simulink model "Simulacion_stepper_2024a"  (R2024a)
settings: Solver=ode4  StartTime=0.0  StopTime=Time_simulation  FixedStep=1/frecuency_simulation  RelTol=1e-3
InitFcn:
  | %%InitFcn();
StopFcn:
  | %%FinishFcn
model workspace (MAT data in the model file):
  Ts_stepper = 0.001
values from neighbouring files (symbols this model uses):
  B = motor_params.B_internal    [bode.m]    (also in current_observer.m = 0.0005; discretizacion.m = [ 1/L, 0; ekf_4_estados.m = params.B; obs_ctrl_back_emf_ext.m = [1/L 0)
  B0 = 3*wn_w - BJ_hat    [Barrido_B.m]    (also in Barrido_J.m; InitFcn.m = 449.962302294)
  B1 = 3*wn_w^2 - B0*BJ_hat    [Barrido_B.m]    (also in Barrido_J.m; InitFcn.m = 64448.3670019)
  B2 = -(J_var/P)*(wn_w^3)    [Barrido_B.m]    (also in Barrido_J.m; InitFcn.m = -0.364323750994)
  B_internal = 1e-4    (= 0.0001)    [InitFcn.m]
  B_var = B_internal* B_factors(k)    [Barrido_B.m]    (also in Barrido_J.m = B_real; InitFcn.m = 0.0001)
  frecuency_simulation = 10e3    (= 10000)    [InitFcn.m]
  I_nom = 1    [InitFcn.m]    (also in salient_motor.m)
  J = motor_params.J_internal    [bode.m]    (also in current_observer.m = 0.008; ekf_4_estados.m = params.J; obs_ctrl_back_emf_ext.m = 0.008; obs_y_contrl_back_emd.m = 0.008)
  J_internal = 4.7/1000000    (= 4.7e-06)    [InitFcn.m]
  J_var = J_real    [Barrido_B.m]    (also in Barrido_J.m = J_internal * J_factors(k); InitFcn.m = 4.7e-06)
  Ke = Kt    [InitFcn.m]    (also in current_observer.m = 0.0055; ekf_4_estados.m = params.Ke; observer.m = Pvec(3); salient_motor.m = 0.0066)
  Ki_d = wd_d*R    (= 3926.99081699)    [InitFcn.m]    (also in bode.m = PI_dq_params.Ki_d_salient)
  Ki_d_salient = wd_d^2*Ld    (= 21491.0635834)    [InitFcn.m]
  Ki_q = wd_q*R    (= 3926.99081699)    [InitFcn.m]    (also in bode.m = PI_dq_params.Ki_q_salient)
  Ki_q_salient = wd_q^2*Lq    (= 7846.33549887)    [InitFcn.m]
  Ki_w = (wn_w^2)*J_var/Kt    [Barrido_B.m]    (also in Barrido_J.m; InitFcn.m; bode.m = PI_MTPA_params.Ki_w)
  Kp_d = wd_d*L    (= 9.42477796077)    [InitFcn.m]    (also in bode.m = PI_dq_params.Kp_d_salient)
  Kp_d_salient = 2*shi_d*wd_d*Ld -R    (= 16.845833313)    [InitFcn.m]
  Kp_q = wd_q*L    (= 9.42477796077)    [InitFcn.m]    (also in bode.m = PI_dq_params.Kp_q_salient)
  Kp_q_salient = 2*shi_q*wd_q*Lq-R    (= 4.56311709936)    [InitFcn.m]
  Kp_w = (2*shi_w*wn_w*J_var)/Kt    [Barrido_B.m]    (also in Barrido_J.m; InitFcn.m; bode.m = PI_MTPA_params.Kp_w)
  Kt = Thold / (sqrt(2) * I_nom)    [InitFcn.m]    (also in current_observer.m = 0.275; ekf_4_estados.m = params.Kt; frecuencia_max.m = 0.33; observer.m = Pvec(4))
  L = 6/1000    (= 0.006)    [InitFcn.m]    (also in current_observer.m = place(A', C', 10*eig(A)).'; desfase.m = lags(k); discretizacion.m = 0.01; frecuencia_max.m)
  Ld = L0 + L2    [Copy_of_PMSM_salient.m]    (also in InitFcn.m = 0.00871; bode.m = motor_params.Ld; ekf_4_estados.m = params.Ld; salient_motor.m = 0.00871)
  Lq = L0 - L2    [Copy_of_PMSM_salient.m]    (also in InitFcn.m = 0.00318; bode.m = motor_params.Lq; ekf_4_estados.m = params.Lq; salient_motor.m = 0.00318)
  N_steps = 360/Step_angle    (= 200)    [InitFcn.m]
  P = N_teeths/2    (= 50)    [InitFcn.m]    (also in bode.m = motor_params.P; ekf_4_estados.m = P_pred; frecuencia_max.m; salient_motor.m)
  Phi = pi/2    (= 1.57079632679)    [InitFcn.m]    (also in ekf_4_estados.m = eye(4) + Ts_eff*A)
  Psi = Kt/P    [InitFcn.m]    (also in bode.m = motor_params.Ke; salient_motor.m = 0.0066)
  R = 2.5    [InitFcn.m]    (also in bode.m = motor_params.R; current_observer.m = 3.4; discretizacion.m = 3.4; ekf_4_estados.m = params.R)
  sample_time = 1/frecuency_simulation    (= 0.0001)    [InitFcn.m]
  Tdm = 18/1000    (= 0.018)    [InitFcn.m]    (also in salient_motor.m)
  Ts_current = 1/f_current    (= 0.0001)    [InitFcn.m]
  Ts_DO = Ts_Wm    (= 0.0001)    [InitFcn.m]
  Ts_ekf = 1/f_ekf    (= 0.0001)    [InitFcn.m]
  Ts_Wm = Ts_current    (= 0.0001)    [InitFcn.m]
  Vdc = 12    [InitFcn.m]    (also in frecuencia_max.m)
undefined symbols (not defined in the file or in its folder): DiscIntNeverNeededParam
libraries: fl_lib x27, nesl_utility x19, spsMosfetLib x16, simulink x8, eeTransforms x4, spsDCVoltageSourceLib x4, spsVoltageMeasurementLib x4, ee_lib x3, slexportprevious_tp74def212_4eb8_4616_a2bc_f4e795655e99 x1, spsTriangleGeneratorLib x1, spspowerguiLib x1
(part 4 of 4)

== matlab function Simulacion_stepper_2024a/Triggered Subsystem7/MATLAB Function ==
  data: Wm input; Vd output; X input; Theta_e input; Ts input; Vdc input; Kp_d input; Ki_d input; Kp_q input; Ki_q input; Ke input; Ld input; Lq input; P input; Vq output; Id output; Iq output; Iq_ref input
function [Vd, Vq, Id, Iq] = PI_dq( ...
    Wm, X, Theta_e, Ts, Vdc, ...
    Kp_d, Ki_d, Kp_q, Ki_q, ...
    Ke, Ld, Lq, P, Iq_ref) % Limpieza de entradas innecesarias

% ================== Estados del Integrador ==================
persistent ek_d u_d ek_q u_q

% Inicialización única
if isempty(u_d)
    u_d = 0; ek_d = 0;
    u_q = 0; ek_q = 0;
end

%% ================== Transformada de Park (abc/ab -> dq) ==================
% X(1) = Ia, X(2) = Ib (Asumiendo motor bifásico/stepper)
Ia = X(1); Ib = X(2);
C = cos(Theta_e); S = sin(Theta_e);

Id =  Ia*C + Ib*S;
Iq = -Ia*S + Ib*C;

%% ================== Desacoples (Feedforward de Corriente) ==================
We = P * Wm;
% V_compensa = Voltaje que el PI no tiene que "esforzarse" en generar
Vdec_d = -Lq * We * Iq;            % Cruce de eje Q sobre D
Vdec_q = (Ke * Wm) + (Ld * We * Id); % Back-EMF + Cruce de eje D sobre Q

%% ================== PI Incremental Eje Q (Torque) ==================
ek_curr_q = Iq_ref - Iq;
k1_q = Kp_q + Ki_q*Ts;
k2_q = -Kp_q;

du_q = k1_q * ek_curr_q + k2_q * ek_q;
u_q  = u_q + du_q;

%% ================== PI Incremental Eje D (Flujo, ref=0) ==================
ek_curr_d = 0 - Id; % Id_ref es siempre 0 para máxima eficiencia
k1_d = Kp_d + Ki_d*Ts;
k2_d = -Kp_d;

du_d = k1_d * ek_curr_d + k2_d * ek_d;
u_d  = u_d + du_d;

%% ================== Salida + Saturación Circular + Anti-Windup ==================
Vd = u_d + Vdec_d;
Vq = u_q + Vdec_q;

Vnorm = sqrt(Vd^2 + Vq^2);

if Vnorm > Vdc
    scale = Vdc / Vnorm;
    Vd = Vd * scale;
    Vq = Vq * scale;
    
    % Anti-windup incremental: "congelamos" la integral restando el exceso
    u_d = Vd - Vdec_d;
    u_q = Vq - Vdec_q;
else
    % Solo actualizamos errores previos si no hubo saturación
    ek_d = ek_curr_d;
    ek_q = ek_curr_q;
end

end

== matlab function Simulacion_stepper_2024a/Triggered Subsystem8/MATLAB Function ==
  data: Wm_ref input; Wm input; Ts input; Kp_w input; Ki_w input; Tl_tdm input; B input; Kt input; Imax input; Iq_ref output
function Iq_ref = PI_speed( ...
        Wm_ref, Wm, Ts, ...
        Kp_w, Ki_w, ...
        Tl_tdm, B, Kt, ...
        Imax)
% ================== Estados del Integrador ==================
persistent ek_w u_w
% Inicialización única al arrancar la simulación
if isempty(u_w)
    u_w  = 0;
    ek_w = 0; 
end

% ================== Feedforward (Modelo de la Planta) ==================
% Torque base necesario para compensar carga y roce viscoso
Iq_ff = (Tl_tdm + B*Wm)/Kt;

% ================== PI incremental ==================
% Error actual
ek_curr = Wm_ref - Wm;

% Constantes del controlador incremental
k1_w = Kp_w + Ki_w*Ts;
k2_w = -Kp_w;

% Cálculo del incremento de control (du) y actualización de la integral (u)
% du = Kp*(ek - ek_prev) + Ki*Ts*ek
du_w = k1_w * ek_curr + k2_w * ek_w;
u_w  = u_w + du_w;

% La referencia final es el aporte del PI + el Feedforward de la planta
Iq_ref = Iq_ff + u_w;

% ================== Saturación con Anti-Windup ==================
if abs(Iq_ref) > Imax
    Iq_ref = sign(Iq_ref) * Imax;
    % Detenemos la integración: restamos el incremento para "congelar" u_w
    u_w = u_w - du_w;
else
    % Solo actualizamos el error previo si no estamos saturados
    % (o puedes actualizarlo siempre, según prefieras el comportamiento del transitorio)
    ek_w = ek_curr;
end

end

== matlab function Simulacion_stepper_2024a/MATLAB Function5 ==
  data: u input; y output
function y = fcn(u)

y = wrap_2pi(u);

== matlab function Simulacion_stepper_2024a/MATLAB Function11 ==
  data: u input; y output
function y = fcn(u)

y = wrap_2pi(u);

== matlab function Simulacion_stepper_2024a/MATLAB Function8 ==
  data: u input; y output
function y = fcn(u)

y = wrap_2pi(u);

== matlab function Simulacion_stepper_2024a/Triggered Subsystem10/MATLAB Function ==
  data: Wm_ref input; Wm input; Ts input; Kp_w input; Ki_w input; Tl_tdm input; B input; Kt input; theta_e input; Tdm input; Imax input; Iq_ref output; Wm_filt_out output
function [Iq_ref,Wm_filt_out] = PI_speed( ...
        Wm_ref, Wm, Ts, ...
        Kp_w, Ki_w, ...
        Tl_tdm, B, Kt, theta_e, Tdm, ...
        Imax)

% ================== Estados Persistentes ==================
% Añadimos Wm_filt para guardar el estado del filtro
persistent ek_w u_w Wm_filt
if isempty(u_w)
    u_w  = 0;
    ek_w = 0; 
    Wm_filt = Wm; % Inicializamos el filtro con el primer valor medido
end

% ================== Filtro Pasabajos (LPF) ==================
% Definimos la frecuencia de corte del filtro (fc). 
% Para un BW de velocidad de 20Hz, un fc de 50-100Hz es ideal.
%  fc = 150; 
%  tau = 1/(2*pi*fc);
% alpha = tau/(tau + Ts); % Coeficiente del filtro
% % 
% % % Aplicamos el filtro a la velocidad medida
%  Wm_f = alpha * Wm_filt + (1 - alpha) * Wm;
%  Wm_filt = Wm_f; % Actualizamos el estado para la próxima iteración

% ================== Feedforward (Modelo de la Planta) ==================
% Es mejor usar la velocidad filtrada para el término viscoso
Iq_ff = (Tl_tdm + B*Wm)/Kt;
Iq_cogging = 0;%% (Tdm * sin(4 * theta_e)) / Kt;
% ================== PI incremental ==================
% El error ahora se calcula con la velocidad FILTRADA
ek_curr = Wm_ref - Wm;

k1_w = Kp_w + Ki_w*Ts;
k2_w = -Kp_w;

du_w = k1_w * ek_curr + k2_w * ek_w;
u_w  = u_w + du_w;

% La referencia final
Iq_ref = -Iq_ff + u_w + Iq_cogging;
Wm_filt_out = Wm_filt;
% ================== Saturación con Anti-Windup ==================
if abs(Iq_ref) > Imax
    Iq_ref = sign(Iq_ref) * Imax;
    u_w = u_w - du_w;
else
    ek_w = ek_curr;
end

end

== matlab function Simulacion_stepper_2024a/Triggered Subsystem2/MATLAB Function ==
  data: U input; x_corr output; X input; Ts input; Ke input; Kt input; R input; J input; Ld input; Lq input; Nr input; B input; Te_est output; Tdm input
function [x_corr, Te_est] = ekf_dq_4states_final(U, X, Ts, Ke, Kt, R, J, Ld, Lq, Nr, B, Tdm)
% =========================================================================
% EKF DE 4 ESTADOS: [Id; Iq; Wm; Th_m]
% =========================================================================
% Entradas:
%   U   = [Vd; Vq]            -> Tensiones de control
%   X   = [Ia; Ib; Theta_e_m] -> Corrientes y Ángulo HFI (Medidos)
%   Ts  = Tiempo de muestreo
% =========================================================================
persistent x_hat P
if isempty(x_hat)
    x_hat = zeros(4,1); 
    % P inicial (4x4)
    P = diag([1e-4, 1e-4, 1e-2, 1e-4]);
end

% -------------------------------------------------------------------------
% 1. TRANSFORMADA DE PARK (Entrada de mediciones)
% -------------------------------------------------------------------------
Ia = X(1); Ib = X(2); The_e_m = X(3);
cos_th = cos(The_e_m);
sin_th = sin(The_e_m);

% Park Directa para obtener corrientes en marco dq medido
Id_m =  Ia * cos_th + Ib * sin_th;
Iq_m = -Ia * sin_th + Ib * cos_th;

Vd_m =  U(1) * cos_th + U(2) * sin_th;
Vq_m = -U(1) * sin_th + U(2) * cos_th;

% -------------------------------------------------------------------------
% 2. PREDICCIÓN (MODELO DE 4 ESTADOS)
% -------------------------------------------------------------------------
Id = x_hat(1); Iq = x_hat(2); Wm = x_hat(3); Th_m = x_hat(4);

% Ecuaciones dinámicas f(x,u)
dId = (Vd_m - R*Id + Nr*Wm*Lq*Iq) / Ld;
dIq = (Vq_m - R*Iq - Nr*Wm*Ld*Id - Ke*Wm) / Lq;
Te  = Kt*Iq + (Ld - Lq)*Id*Iq; % Torque total
% Nota: Aquí eliminamos Tx. El torque de carga ahora se trata como ruido de proceso.
dWm = (Te - B*Wm - Tdm*sin(4*Nr*Th_m)) / J; 
dTh = Wm;

% Predicción de estado (Integración de Euler)
x_pred = x_hat + Ts * [dId; dIq; dWm; dTh];
x_pred(4) = wrap_pi(x_pred(4));

% -------------------------------------------------------------------------
% 3. LINEALIZACIÓN (JACOBIANO A DE 4x4)
% -------------------------------------------------------------------------
A = [ -R/Ld,                Nr*Wm*Lq/Ld,         Nr*Lq*Iq/Ld,         0;
     -Nr*Wm*Ld/Lq,         -R/Lq,               -(Nr*Ld*Id + Ke)/Lq,  0;
      (Ld-Lq)*Iq/J,     (Kt + Nr*(Ld-Lq)*Id)/J, -B/J,              0;
      0,                   0,                   1,                    0];
    
Phi = eye(4) + A*Ts;

% Covarianza del proceso Qk (4x4)
% Al no estimar Tx, es vital que Qk(3,3) sea un poco más alto para absorber
% las variaciones de carga como incertidumbre en la velocidad.
Qk = diag([1e-6, 1e-6, 1e-6, 1e-10]); 
P_pred = Phi * P * Phi' + Qk;

% -------------------------------------------------------------------------
% 4. CORRECCIÓN (INNOVACIÓN Y GANANCIA)
% -------------------------------------------------------------------------
% Matriz de observación Ck (Medimos Id, Iq y Theta_e_m -> Nr * Th_m)
Ck = [1 0 0 0;
      0 1 0 0;
      0 0 0 Nr]; 

% Ruido de medición
Rk = diag([1e-3, 1e-3, 1e-8]);

y_meas = [Id_m; Iq_m; The_e_m];
y_pred = [x_pred(1); x_pred(2); Nr * x_pred(4)];

innov = y_meas - y_pred;
innov(3) = wrap_pi(innov(3));

% Ganancia de Kalman
Sk = Ck * P_pred * Ck' + Rk;
Lk = (P_pred * Ck') / Sk; % Lk es ahora de 4x3

% Actualización de estado y covarianza
x_corr = x_pred + Lk * innov;
x_corr(4) = wrap_pi(x_corr(4));

P = (eye(4) - Lk*Ck) * P_pred;
P = 0.5 * (P + P'); % Asegurar simetría

% -------------------------------------------------------------------------
% 5. PERSISTENCIA Y SALIDAS
% -------------------------------------------------------------------------
x_hat = x_corr;
Te_est = Kt*x_corr(2) + (Ld-Lq)*x_corr(1)*x_corr(2);

end

function out = wrap_pi(in)
    out = atan2(sin(in), cos(in));
end

== matlab function Simulacion_stepper_2024a/Triggered Subsystem2/MATLAB Function1 ==
  data: U input; x_corr output; X input; Ts input; Kt input; R input; J input; L input; Nr input; B input; Ke input
function x_corr = ekf_5var(U,X,Ts,Kt,R,J,L,Nr,B,Ke)
persistent x_hat P x_pred
%%  x_hat son los estados predichos
%%  x_corr es la salida corregida
%%  P_pre ó Sum_less es la covarianza predicha
%%  P ó sum_more es la covarianza
%%  Rk ó sum_v es la covarianza de incertidumbre del sensor




 %%Iniciamos calculando X_hat[k-1]
 if isempty(x_hat)
     x_hat = zeros(5,1);
     P = diag([1e-4 1e-4 1e-6 1e-10 1e-4]);
     x_corr = zeros(5,1);
     x_pred = zeros(5,1);


 end

Qk = diag([1e-4 1e-4 1e-4 1e-10 1e-6]);
Rk = diag([5e-4 5e-4]);   % ruido de medición

%%1A
%%Predicción
Ia = x_hat(1);
Ib = x_hat(2);
Wm = x_hat(3);
Th_m = x_hat(4);
Tx = x_hat(5);

Th_e = Nr*Th_m;
S = sin(Th_e);
C = cos(Th_e);

Va = U(1);
Vb = U(2);

dx = zeros(5,1);
dx(1) = (Va - R*Ia + Ke*Wm*S)/L;
dx(2) = (Vb - R*Ib - Ke*Wm*C)/L;
dx(3) = (Kt*(Ib*C-Ia*S) -Tx)/J;
dx(4) = Wm;
dx(5) = 0;
x_pred = x_hat + Ts*dx;
x_pred(4) = wrap_2pi(x_pred(4));

%%Calculamos el jacobiano
RL = R/L;
uno = Ke*S;
dos = Ke*C;

A = [-RL 0   (uno/L) (dos*Nr*Wm/L) 0;
 0  -RL   -dos/L    uno*Nr*Wm/L  0;
 -uno/J dos/J -1/J -Kt*Nr*(Ia*C+Ib*S)/J -1/J;
 0 0 1 0 0;
 0 0 0 0 0];

A_hat = eye(5) + Ts*A;
A_hat_T = transpose(A_hat);

%%1B COVARIANZA PREDICHA
P_pred = A_hat * P * A_hat_T + Qk; 


%%1C PREDECIMOS LA SALIDA DEL SISTEMA
Ck = [1 0 0 0 0;
      0 1 0 0 0];
Ck_T = transpose(Ck);
y_pred = Ck*x_pred;

%%2A calculamos la matriz Lk
%%Lk = P_pred *Ck_T * inv(Ck*P_pred*Ck_T + sum_v)
Sk = Ck*P_pred*Ck_T + Rk;
Lk = P_pred * Ck_T /Sk;

%%2B Actualizamos los estados estados corregidos en función de L


y_meas = [X(1);X(2)];

innov = y_meas - y_pred;
x_corr = x_pred + Lk*(innov);
x_corr(4) = wrap_2pi(x_corr(4));
%%actualizamos la covarianza y guardamos el estado
x_hat = x_corr;
Lk_T = transpose(Lk);
P = P_pred - Lk*Sk*Lk_T;
P_T = transpose(P);
P = 0.5 * (P + P_T);

== matlab function Simulacion_stepper_2024a/Triggered Subsystem2/MATLAB Function2 ==
  data: U input size=2; x_corr output; Y input size=2; Ts input; Kt input; R input; J input; L input; Nr input; B input
function x_corr = SPKF_4var(U,Y,Ts,Kt,R,J,L,Nr,B)
persistent x_hat P  alpham alphac Qk Rk h
%%  x_hat son los estados predichos
%%  x_corr es la salida corregida
%%  P_pre ó Sum_less es la covarianza predicha
%%  P ó sum_more es la covarianza
%%  Rk ó sum_v es la covarianza de incertidumbre del sensor


Nx = 4; %%Números de estados
Nw = 4; %% Incertidumbres de estado
Ny = 2; %% Incertidumbre de mediciones
Na = Nx+Nw+Ny;


%%Los métodos de sigma-point pueden diferir al utilizar las variables
%%alpha. Existen 2 métodos:

%% Método |    Sigma       |     alpha_m_0      | alpha_m_k         |           alpha_c_0               | alpha_c_k |
%% UKF    | sqrt(L+lambda) |  lambda/(L+Lambda) | 1/(2*(L+Lambda))  | alpha_m_0 + (1-alpha^2 + betha)   | alpha_m_k |
%% CDKF   |    h           |   (h^2 - L)/h^2    |  1/(2*h^2)        | alpha_m_0                         | alpha_m_k |
 %%Iniciamos calculando X_hat[k-1]
 if isempty(x_hat)
    
     %%Utilizamos el CDKF, con h = sqrt(Nxa); 
        x_hat = zeros(Nx,1);
        h =sqrt(Na);
        alpham = ones(2*Na+1,1) * (1/(2*h^2));
        alpham(1) = (h^2 - Na)/(h^2);   % peso del sigma central
        alphac = alpham;             
     %%Valores de covarianza
     P = diag([1e-2 1e-2 1e-6 1e-12 ]);
     Qk = diag([1e-2 1e-2 1e-8 1e-12 ]);
     Rk = [1e-4 0; 0 1e-4];
 end
    
     x_corr = zeros(Nx,1);
     x_pred = zeros(Nx,1);
     x_hat_a = zeros(Na,1);
     X_minus = zeros(Nx,2*Na+1);
     Y_minus = zeros(Ny,2*Na+1);
%%Ciclo de 2*Na+1
%%Aun que deberiamos hacer un ciclo for, en matlab se hace solo asi que no
%%es necesario

%% 1A-I Creamos el vector de estados extendidos
x_hat_a = [x_hat;zeros(Nw,1);zeros(Ny,1)]; 


%% 1A-II Conseguimos el factor de cholesky


%%Creamos la matriz de covarianza extendidas, el cual es de la forma
%%             [P   0    0]
%%     P_a =   [0   Qk   0]
%%             [0   0   Rk]

P_a = blkdiag(P,Qk,Rk);
Sa = chol(P_a,"lower");

%% 1A-III generamos los sigma points
%% Queda de la forma [x_hat_a, x_hat_a + h*S,x_hat_a - h*S] (Por eso es 2*Nxa+1 = N)
%% Al usar x_a x_a(:,ones(1,Na)) creamos una matriz de la forma [x_a,x_a...x_a], que es de tamaño (Na)x(2*Na+1)
%% Posteriormente, se le suma un vector de [0,+h*S,-h*S]
%% Cómo S es del tamaño (Nxa)x(Nxa), el total es de (2*Na+1 = N)
X =  x_hat_a(:,ones(1,2*Na+1)) + h*[zeros(Na,1), Sa, -Sa];

%% 1A-IV Calculamos las ecuaciones de estado
Va = U(1);
Vb = U(2);


for k=1:2*Na+1

  % --- separar estado, ruido de proceso y ruido de medición ---


xk = X(1:Nx,k);                     % [Ia; Ib; Wm; Th_m]
wk = X(Nx+1 : Nx+Nw,k);             % ruido de proceso (4x1)
vk = X(Nx+Nw+1 : end,k);            % ruido de medición (2x1)    

Ia = xk(1);
Ib = xk(2);
Wm = xk(3);
Th_m = xk(4);

Th_e = Nr*Th_m;
S = sin(Th_e);
C = cos(Th_e);


dx1 = (Va - R*Ia + Kt*Wm*S)/L;
dx2 = (Vb - R*Ib - Kt*Wm*C)/L;
dx3 = (Kt*(Ib*C-Ia*S)-B*Wm)/J;
dx4 = Wm;

%Calculamos el paso siguiente mediante euler
%% X_minus corresponde a la matriz que contiene todos los sigma-points distribuidos en los estados del sistema no-extendido (Nx)x(Na)
X_minus(1,k) = Ia + Ts*dx1+ wk(1);
X_minus(2,k) = Ib + Ts*dx2 + wk(2);
X_minus(3,k) = Wm + Ts*dx3 + wk(3);
X_minus(4,k) = Th_m + Ts*dx4 + wk(4);
%%X_minus(4,k) = wrap_2pi(X_minus(4,k));

Y_minus(1,k) = X_minus(1,k) + vk(1);
Y_minus(2,k) = X_minus(2,k) + vk(2);

end
%% 1B Reconstrucción de la media
%% Esta matriz contiene la media de todos los estados. (Nx)x(1)
x_pred = X_minus*alpham;
y_pred = Y_minus*alpham;
%%  Reconstrucción de la covarianza

%% Acá lo que hacemos es copiar la media N veces, para poder realizar la resta.
%%Pero realmente debería ser un for de [Xs(i,k)= X_minus(i,k) - x_pred(i)],
%%dónde K es cada variable de estado (Nx)
%% Xs es una matriz de desviación respecto a la media. Es necesario para construir la covarianza P
Xs = X_minus - x_pred(:,ones([1 2*Na+1])); 
Ys = Y_minus - y_pred(:,ones([1 2*Na+1]));

Xs_T = transpose(Xs);
Ys_T = transpose(Ys);
%%Calculamos la matriz de covarianza, pero hay que considerar que como
%%diag(alphac) es una matriz llena de diagonales, uno puede reducir la
%%cantidad de cómputo.
P_pred = Xs*diag(alphac)*Xs_T;
Pyy = Ys* diag(alphac)* Ys_T;
Pxy = Xs*diag(alphac)*Ys_T;
Lk = Pxy/Pyy;
Lk_T = transpose(Lk);
%% 2B Leemos la medición y actualizamos
x_corr = x_pred + Lk*(Y - y_pred);
x_corr(4) = wrap_2pi(x_corr(4));
%%Guardamos los valores de x_hat para mantenerlos
x_hat = x_corr; 
%% 2C Actualizamos la covarianza
P = P_pred - Lk*Pyy*Lk_T;
P_T = transpose(P);
P = 0.5 * (P + P_T);

== matlab function Simulacion_stepper_2024a/Triggered Subsystem2/MATLAB Function3 ==
  data: U input size=2; x_corr output; Y input size=2; Ts input; Kt input; R input; J input; L input; Nr input; B input
function x_corr = SPKF_5var(U,Y,Ts,Kt,R,J,L,Nr,B)
persistent x_hat P x_pred alpham alphac Qk Rk h
%%  x_hat son los estados predichos
%%  x_corr es la salida corregida
%%  P_pre ó Sum_less es la covarianza predicha
%%  P ó sum_more es la covarianza
%%  Rk ó sum_v es la covarianza de incertidumbre del sensor


Nx = 5; %%Números de estados
Nw = 5; %% Incertidumbres de estado
Ny = 2; %% Incertidumbre de mediciones
Na = Nx+Nw+Ny;


%%Los métodos de sigma-point pueden diferir al utilizar las variables
%%alpha. Existen 2 métodos:

%% Método |    Sigma       |     alpha_m_0      | alpha_m_k         |           alpha_c_0               | alpha_c_k |
%% UKF    | sqrt(L+lambda) |  lambda/(L+Lambda) | 1/(2*(L+Lambda))  | alpha_m_0 + (1-alpha^2 + betha)   | alpha_m_k |
%% CDKF   |    h           |   (h^2 - L)/h^2    |  1/(2*h^2)        | alpha_m_0                         | alpha_m_k |
 %%Iniciamos calculando X_hat[k-1]
 if isempty(x_hat)
    
     %%Utilizamos el CDKF, con h = sqrt(Nxa); 
        x_hat = zeros(Nx,1);
        h =sqrt(Na);
        alpham = ones(2*Na+1,1) * (1/(2*h^2));
        alpham(1) = (h^2 - Na)/(h^2);   % peso del sigma central
        alphac = alpham;             
     %%Valores de covarianza
     P = diag([1e-2 1e-2 1e-4 1e-8 1e-12]);
     Qk = diag([1e-2 1e-2 1e-6 1e-8 1e-12]);
     Rk = [1e-4 0; 0 1e-4];
 end
    
     x_corr = zeros(Nx,1);
     x_pred = zeros(Nx,1);
     x_hat_a = zeros(Na,1);
     X_minus = zeros(Nx,2*Na+1);
     Y_minus = zeros(Ny,2*Na+1);
%%Ciclo de 2*Na+1
%%Aun que deberiamos hacer un ciclo for, en matlab se hace solo asi que no
%%es necesario

%% 1A-I Creamos el vector de estados extendidos
x_hat_a = [x_hat;zeros(Nw,1);zeros(Ny,1)]; 


%% 1A-II Conseguimos el factor de cholesky


%%Creamos la matriz de covarianza extendidas, el cual es de la forma
%%             [P   0    0]
%%     P_a =   [0   Qk   0]
%%             [0   0   Rk]

P_a = blkdiag(P,Qk,Rk);
Sa = chol(P_a,"lower");

%% 1A-III generamos los sigma points
%% Queda de la forma [x_hat_a, x_hat_a + h*S,x_hat_a - h*S] (Por eso es 2*Nxa+1 = N)
%% Al usar x_a x_a(:,ones(1,Na)) creamos una matriz de la forma [x_a,x_a...x_a], que es de tamaño (Na)x(2*Na+1)
%% Posteriormente, se le suma un vector de [0,+h*S,-h*S]
%% Cómo S es del tamaño (Nxa)x(Nxa), el total es de (2*Na+1 = N)
X =  x_hat_a(:,ones(1,2*Na+1)) + h*[zeros(Na,1), Sa, -Sa];

%% 1A-IV Calculamos las ecuaciones de estado
Va = U(1);
Vb = U(2);


for k=1:2*Na+1

  % --- separar estado, ruido de proceso y ruido de medición ---


xk = X(1:Nx,k);                     % [Ia; Ib; Wm; Th_m]
wk = X(Nx+1 : Nx+Nw,k);             % ruido de proceso (4x1)
vk = X(Nx+Nw+1 : end,k);            % ruido de medición (2x1)    

Ia = xk(1);
Ib = xk(2);
Wm = xk(3);
Th_m = xk(4);
Tx = xk(5);

Th_e = Nr*Th_m;
S = sin(Th_e);
C = cos(Th_e);


dx1 = (Va - R*Ia + Kt*Wm*S)/L;
dx2 = (Vb - R*Ib - Kt*Wm*C)/L;
dx3 = (Kt*(Ib*C-Ia*S)-B*Wm - Tx)/J;
dx4 = Wm;
dTx = 0;

%Calculamos el paso siguiente mediante euler
%% X_minus corresponde a la matriz que contiene todos los sigma-points distribuidos en los estados del sistema no-extendido (Nx)x(Na)
X_minus(1,k) = Ia + Ts*dx1+ wk(1);
X_minus(2,k) = Ib + Ts*dx2 + wk(2);
X_minus(3,k) = Wm + Ts*dx3 + wk(3);
X_minus(4,k) = Th_m + Ts*dx4 + wk(4);
X_minus(4,k) = wrap_2pi(X_minus(4,k));
X_minus(5,k) = Tx + Ts*dTx + wk(5);

Y_minus(1,k) = X_minus(1,k) + vk(1);
Y_minus(2,k) = X_minus(2,k) + vk(2);

end
%% 1B Reconstrucción de la media
%% Esta matriz contiene la media de todos los estados. (Nx)x(1)
x_pred = X_minus*alpham;
y_pred = Y_minus*alpham;
%%  Reconstrucción de la covarianza

%% Acá lo que hacemos es copiar la media N veces, para poder realizar la resta.
%%Pero realmente debería ser un for de [Xs(i,k)= X_minus(i,k) - x_pred(i)],
%%dónde K es cada variable de estado (Nx)
%% Xs es una matriz de desviación respecto a la media. Es necesario para construir la covarianza P
Xs = X_minus - x_pred(:,ones([1 2*Na+1])); 
Ys = Y_minus - y_pred(:,ones([1 2*Na+1]));

Xs_T = transpose(Xs);
Ys_T = transpose(Ys);
%%Calculamos la matriz de covarianza, pero hay que considerar que como
%%diag(alphac) es una matriz llena de diagonales, uno puede reducir la
%%cantidad de cómputo.
P_pred = Xs*diag(alphac)*Xs_T;
Pyy = Ys* diag(alphac)* Ys_T;
Pxy = Xs*diag(alphac)*Ys_T;
Lk = Pxy/Pyy;
Lk_T = transpose(Lk);
%% 2B Leemos la medición y actualizamos
x_corr = x_pred + Lk*(Y - y_pred);
x_corr(4) = wrap_2pi(x_corr(4));
%%Guardamos los valores de x_hat para mantenerlos
x_hat = x_corr; 
%% 2C Actualizamos la covarianza
P = P_pred - Lk*Pyy*Lk_T;
P_T = transpose(P);
P = 0.5 * (P + P_T);

== matlab function Simulacion_stepper_2024a/MATLAB Function9 ==
  data: u input; y output
function y = fcn(u)

y = wrap_2pi(u);

== matlab function Simulacion_stepper_2024a/MATLAB Function10 ==
  data: u input; y output
function y = fcn(u)

y = wrap_2pi(u);

== matlab function Simulacion_stepper_2024a/Triggered Subsystem4/MATLAB Function ==
  data: Wm input; x_corr output; Iq input; Ts input; Kt input; J input
function x_corr = ekf_2var(Wm,Iq,Ts,Kt,J)
persistent x_hat P x_pred
%%  x_hat son los estados predichos
%%  x_corr es la salida corregida
%%  P_pre ó Sum_less es la covarianza predicha
%%  P ó sum_more es la covarianza
%%  Rk ó sum_v es la covarianza de incertidumbre del sensor




 %%Iniciamos calculando X_hat[k-1]
 if isempty(x_hat)
     x_hat = zeros(2,1);
     P = diag([1e-5 1e-3 ]);
     x_corr = zeros(2,1);
     x_pred = zeros(2,1);


 end

Qk = diag([1e-2 5e-7]);
Rk = diag(5e-1);   % ruido de medición

%%1A
%%Predicción

Wm = x_hat(1);
Tx = x_hat(2);


Te = Iq*Kt;

dx = zeros(2,1);
dx(1) = (Te - Tx)/J;
dx(2) = 0;

x_pred = x_hat + Ts*dx;




A = [0 -1/J; 0 0];

% A_hat = eye(4) + Ts*A;
A_hat = expm(A*Ts);
A_hat_T = transpose(A_hat);

%%1B COVARIANZA PREDICHA
P_pred = A_hat * P * A_hat_T + Qk; 


%%1C PREDECIMOS LA SALIDA DEL SISTEMA
Ck = [1 0];
Ck_T = transpose(Ck);
y_pred = Ck*x_pred;

%%2A calculamos la matriz Lk
%%Lk = P_pred *Ck_T * inv(Ck*P_pred*Ck_T + sum_v)
Sk = Ck*P_pred*Ck_T + Rk;
Lk = P_pred * Ck_T /Sk;

%%2B Actualizamos los estados estados corregidos en función de L


y_meas = Wm;

innov = y_meas - y_pred;
x_corr = x_pred + Lk*(innov);

%%actualizamos la covarianza y guardamos el estado
x_hat = x_corr;
Lk_T = transpose(Lk);
P = P_pred - Lk*Sk*Lk_T;
P_T = transpose(P);
P = 0.5 * (P + P_T);

== matlab function Simulacion_stepper_2024a/MATLAB Function12 ==
  data: u input; y output
function y = fcn(u)

y = wrap_2pi(u);

== matlab function Simulacion_stepper_2024a/Triggered Subsystem4/MATLAB Function1 ==
  data: theta_EKF input; Iq_obs input; Ts input; Kt input; np input; J input; theta_hat output; omega_hat output; d_hat output; B input; beta0 input; beta1 input; beta2 input
function [theta_hat, omega_hat, d_hat] = DO_paper( ...
        theta_EKF,Iq_obs, Ts, Kt, np, J, B, beta0, beta1, beta2)

% -----------------------------------------------------------
% Disturbance Observer (Linear DO) from Eq. (36) of the paper:
%   "Simultaneous State and Disturbance Estimation for 
%         Sensorless PMSM Control"
%
% Inputs:
%   theta_EKF  = \hatθ_e^E[k] (EKF estimated electrical angle)
%   omega_EKF  = \hatω_e^E[k] (EKF estimated electrical speed)
%   iq         = i_q(k)
%   Ts         = sampling period
%   Kt         = torque constant in dq model (Kτ)
%   np         = pole pairs
%   J          = inertia
%   B          = viscous friction
%   beta0,beta1,beta2 = DO gains
%
% Outputs:
%   theta_hat = \hatθ_e[k]
%   omega_hat = \hatω_e[k]
%   d_hat     = \hat d[k]  (estimated load torque T_L)
% -----------------------------------------------------------

persistent theta omega d

if isempty(theta)
    theta = 0;
    omega = 0;
    d     = 0;
end

%% ============================
%  (1) Error term Eq. (36)
% =============================
% e0 = θ_E^E[k] − θ̂_e[k−1]
e0 = wrap_2pi(theta_EKF - theta);

%% ============================
%  (2) Angle update Eq. (36)
% ============================
theta_hat = theta + Ts*( omega + beta0 * e0 );
theta_hat = wrapTo2Pi(theta_hat);

%% ============================
%  (3) Speed update Eq. (36)
% ============================
omega_hat = omega ...
    + Ts * ( Kt * Iq_obs/J ...
           - (np/J) * d ...
           - (B/J) * omega ...
           + beta1 * e0 );

%% ============================
%  (4) Disturbance update Eq. (36)
% ============================
d_hat = d + Ts * beta2 * e0;

%% ============================
%  (5) Save states
% ============================
theta = theta_hat;
omega = omega_hat;
d     = d_hat;

end

== matlab function Simulacion_stepper_2024a/MATLAB Function14 ==
  data: u input; y output
function y = fcn(u)

y = wrap_2pi(u);

== matlab function Simulacion_stepper_2024a/Triggered Subsystem3/MATLAB Function ==
  data: Wm input; x_corr output; Iq input; Ts input; Kt input; J input
function x_corr = ekf_2var(Wm,Iq,Ts,Kt,J)
persistent x_hat P x_pred
%%  x_hat son los estados predichos
%%  x_corr es la salida corregida
%%  P_pre ó Sum_less es la covarianza predicha
%%  P ó sum_more es la covarianza
%%  Rk ó sum_v es la covarianza de incertidumbre del sensor




 %%Iniciamos calculando X_hat[k-1]
 if isempty(x_hat)
     x_hat = zeros(2,1);
     P = diag([1e-5 1e-3 ]);
     x_corr = zeros(2,1);
     x_pred = zeros(2,1);


 end

Qk = diag([1e-2 5e-7]);
Rk = diag(5e-1);   % ruido de medición

%%1A
%%Predicción

Wm = x_hat(1);
Tx = x_hat(2);


Te = Iq*Kt;

dx = zeros(2,1);
dx(1) = (Te - Tx)/J;
dx(2) = 0;

x_pred = x_hat + Ts*dx;




A = [0 -1/J; 0 0];

% A_hat = eye(4) + Ts*A;
A_hat = expm(A*Ts);
A_hat_T = transpose(A_hat);

%%1B COVARIANZA PREDICHA
P_pred = A_hat * P * A_hat_T + Qk; 


%%1C PREDECIMOS LA SALIDA DEL SISTEMA
Ck = [1 0];
Ck_T = transpose(Ck);
y_pred = Ck*x_pred;

%%2A calculamos la matriz Lk
%%Lk = P_pred *Ck_T * inv(Ck*P_pred*Ck_T + sum_v)
Sk = Ck*P_pred*Ck_T + Rk;
Lk = P_pred * Ck_T /Sk;

%%2B Actualizamos los estados estados corregidos en función de L


y_meas = Wm;

innov = y_meas - y_pred;
x_corr = x_pred + Lk*(innov);

%%actualizamos la covarianza y guardamos el estado
x_hat = x_corr;
Lk_T = transpose(Lk);
P = P_pred - Lk*Sk*Lk_T;
P_T = transpose(P);
P = 0.5 * (P + P_T);

== matlab function Simulacion_stepper_2024a/Triggered Subsystem9/MATLAB Function ==
  data: Wm input; Vd output; X input; Theta_e input; Ts input; Vdc input; Kp_d input; Ki_d input; Kp_q input; Ki_q input; Psi input; Ld input; Lq input; P input; Vq output; Iq_ref_req input; Valpha output; Vbetha output
function [Vd, Vq,Valpha,Vbetha] = PI_dq_vectorial_fixed(Wm, X, Theta_e, Ts, Vdc, ...
                                           Kp_d, Ki_d, Kp_q, Ki_q, ...
                                           Psi, Ld, Lq, P, Iq_ref_req)
% Parámetros internos
I_max = sqrt(2); 
persistent v_int_d v_int_q Id_filt Iq_filt
if isempty(v_int_d)
    v_int_d = 0; 
    v_int_q = 0; 
    Id_filt = 0;
    Iq_filt = 0;
end

% 
%  fc_d = 1200; 
%  tau_d = 1/(2*pi*fc_d);
% alpha_d = tau_d/(tau_d + Ts); % Coeficiente del filtro
% 
%  fc_q = 600; 
%  tau_q = 1/(2*pi*fc_q);
% alpha_q = tau_q/(tau_q + Ts); % Coeficiente del filtro
%% 1. Transformada de Park
Id = X(1); Iq = X(2);





% % Aplicamos el filtro a la velocidad medida
 % Id_f = alpha_d * Id_filt + (1 - alpha_d) * Id;
 % Id_filt = Id_f; % Actualizamos el estado para la próxima iteración
 % 
 % % % Aplicamos el filtro a la velocidad medida
 % Iq_f = alpha_q * Iq_filt + (1 - alpha_q) * Iq;
 % Iq_filt = Iq_f; % Actualizamos el estado para la próxima iteración
%% 2. Referencias con Saturación Vectorial
Id_ref = 0; 
Iq_limit = sqrt(max(0, I_max^2 - Id_ref^2)); 
Iq_ref = max(-Iq_limit, min(Iq_limit, Iq_ref_req));

%% 3. Errores y Desacoples
err_d = Id_ref - Id;
err_q = Iq_ref - Iq;
We = P * Wm; 

% Términos de Desacople
V_cross_d = -We * Lq * Iq; 
V_cross_q =  We * Ld * Id + We * Psi; 

%% 4. Cálculo de Voltaje Base (PI + Feedforward)
Vd_pre = Kp_d * err_d + v_int_d + V_cross_d;
Vq_pre = Kp_q * err_q + v_int_q + V_cross_q;

%% 5. Protección de Corriente y Saturación de Voltaje
I_mag_real = sqrt(Id^2 + Iq^2);
limit_V = Vdc;

% Si la corriente real excede el límite de seguridad (1.2A)
if I_mag_real > 1.2
    limit_V = Vdc * (1.0 / I_mag_real);
end

% Saturación Circular de Voltaje
V_mag = sqrt(Vd_pre^2 + Vq_pre^2);

if V_mag > limit_V
    Vd = (Vd_pre / V_mag) * limit_V;
    Vq = (Vq_pre / V_mag) * limit_V;
    sat_active = true;
else
    Vd = Vd_pre;
    Vq = Vq_pre;
    sat_active = false;
end

%% 6. Anti-Windup (Clamping)
if ~sat_active || (sign(err_d) ~= sign(v_int_d))
    v_int_d = v_int_d + Ki_d * Ts * err_d;
end
if ~sat_active || (sign(err_q) ~= sign(v_int_q))
    v_int_q = v_int_q + Ki_q * Ts * err_q;
end



%% 7. Transformada Inversa de Park (Salida a Marco Estacionario)
% Usamos el MISMO ángulo desfasado que en la entrada para mantener la coherencia
Valpha = Vd * cos(Theta_e) - Vq *sin(Theta_e);
Vbetha = Vd * sin(Theta_e) + Vq *cos(Theta_e);
end

== matlab function Simulacion_stepper_2024a/MATLAB Function1 ==
  data: u input; y output
function y = fcn(u)

y = wrap_2pi(u);

== matlab function Simulacion_stepper_2024a/MATLAB Function2 ==
  data: u input; y output
function y = fcn(u)

y = wrap_2pi(u);

== matlab function Simulacion_stepper_2024a/MATLAB Function3 ==
  data: u input; y output
function y = fcn(u)

y = wrap_2pi(u);

== matlab function Simulacion_stepper_2024a/Triggered Subsystem1/MATLAB Function ==
  data: U input; x_corr output; X input; Ts input; Ke input; Kt input; R input; J input; Ld input; Lq input; Nr input; N_steps input; B input; d_hat output; Tdtm input; beta0 input; beta1 input; beta2 input
function [x_corr, d_hat] = ekf_dq_4states_final(U, X, Ts, Ke, Kt, R, J, Ld, Lq, Nr, N_steps,B, Tdtm,beta0,beta1,beta2)
% =========================================================================
% EKF DE 4 ESTADOS: [Id; Iq; Wm; Th_m]
% =========================================================================
% Entradas:
%   U   = [Vd; Vq]            -> Tensiones de control
%   X   = [Ia; Ib; Theta_e_m] -> Corrientes y Ángulo HFI (Medidos)
%   Ts  = Tiempo de muestreo
% =========================================================================
persistent x_hat P d_do theta_do omega_do 
if isempty(x_hat)
    x_hat = zeros(4,1); 
    % P inicial (4x4)
    P = diag([1e-4, 1e-4, 1e-2, 1e-4]);
    theta_do = 0;
    omega_do = 0;
   
end

% -------------------------------------------------------------------------
% 1. TRANSFORMADA DE PARK (Entrada de mediciones)
% -------------------------------------------------------------------------
Ia = X(1); Ib = X(2); The_e_m = X(3);
cos_th = cos(The_e_m);
sin_th = sin(The_e_m);

% Park Directa para obtener corrientes en marco dq medido
Id_m =  Ia * cos_th + Ib * sin_th;
Iq_m = -Ia * sin_th + Ib * cos_th;

Vd_m =  U(1) * cos_th + U(2) * sin_th;
Vq_m = -U(1) * sin_th + U(2) * cos_th;

% -------------------------------------------------------------------------
% 2. PREDICCIÓN (MODELO DE 4 ESTADOS)
% -------------------------------------------------------------------------
Id = x_hat(1); Iq = x_hat(2); Wm = x_hat(3); Th_m = x_hat(4);


% Ecuaciones dinámicas f(x,u)
dId = (Vd_m - R*Id + Nr*Wm*Lq*Iq) / Ld;
dIq = (Vq_m - R*Iq - Nr*Wm*Ld*Id - Ke*Wm) / Lq;
Te  = Kt*Iq + Nr*(Ld - Lq)*Id*Iq; % Torque total
% Nota: Aquí eliminamos Tx. El torque de carga ahora se trata como ruido de proceso.
dWm = (Te - B*Wm  - d_do ) / J; 
dTh = Wm;

% Predicción de estado (Integración de Euler)
x_pred = x_hat + Ts * [dId; dIq; dWm; dTh];
x_pred(4) = wrap_pi(x_pred(4));

% -------------------------------------------------------------------------
% 3. LINEALIZACIÓN (JACOBIANO A DE 4x4)
% -------------------------------------------------------------------------




A = [ -R/Ld,                Nr*Wm*Lq/Ld,         Nr*Lq*Iq/Ld,         0;
     -Nr*Wm*Ld/Lq,         -R/Lq,               -(Nr*Ld*Id + Ke)/Lq,  0;
      (Ld-Lq)*Iq/J,     (Kt + Nr*(Ld-Lq)*Id)/J, -B/J,              0;
      0,                   0,                   1,                    0];
    
Phi = eye(4) + A*Ts;

% Covarianza del proceso Qk (4x4)
% Al no estimar Tx, es vital que Qk(3,3) sea un poco más alto para absorber
% las variaciones de carga como incertidumbre en la velocidad.
Qk = diag([1e-6, 1e-6, 1e-6, 1e-10]); 
P_pred = Phi * P * Phi' + Qk;

% -------------------------------------------------------------------------
% 4. CORRECCIÓN (INNOVACIÓN Y GANANCIA)
% -------------------------------------------------------------------------
% Matriz de observación Ck (Medimos Id, Iq y Theta_e_m -> Nr * Th_m)
Ck = [1 0 0 0;
      0 1 0 0;
      0 0 0 Nr]; 

% Ruido de medición
Rk = diag([1e-3, 1e-3, 1e-8]);

y_meas = [Id_m; Iq_m; The_e_m];
y_pred = [x_pred(1); x_pred(2); Nr * x_pred(4)];

innov = y_meas - y_pred;
innov(3) = wrap_pi(innov(3));

% Ganancia de Kalman
Sk = Ck * P_pred * Ck' + Rk;
Lk = (P_pred * Ck') / Sk; % Lk es ahora de 4x3

% Actualización de estado y covarianza
x_corr = x_pred + Lk * innov;
x_corr(4) = wrap_pi(x_corr(4));

P = (eye(4) - Lk*Ck) * P_pred;
P = 0.5 * (P + P'); % Asegurar simetría

% -------------------------------------------------------------------------
% 5. Disturbed observer
% -------------------------------------------------------------------------


theta_ekf = x_corr(4);

e0 = wrap_pi(theta_ekf - theta_do);

Te_obs = Kt*Iq + (Ld-Lq)*Id_m*Iq_m;

theta_do = theta_do + Ts*(omega_do + beta0*e0);
theta_do = wrap_pi(theta_do);


Tdm_hat = Tdtm*sin(N_steps*theta_ekf/P);

omega_do = omega_do + Ts*((Te_obs - d_do - Tdm_hat - B*omega_do)/J + beta1*e0);

d_do = d_do + Ts*beta2*e0;

% -------------------------------------------------------------------------
% 6. PERSISTENCIA Y SALIDAS
% -------------------------------------------------------------------------
x_hat = x_corr;
d_hat = d_do + Tdm_hat;
end

function out = wrap_pi(in)
    out = atan2(sin(in), cos(in));
end
